simulink model "unknown_case"  (R2021a)
settings: Solver=VariableStepAuto  StartTime=0.0  StopTime=20.0  RelTol=1e-3
libraries: simulink x1
settings Model: Creator=tejal  LastModifiedBy=tejal

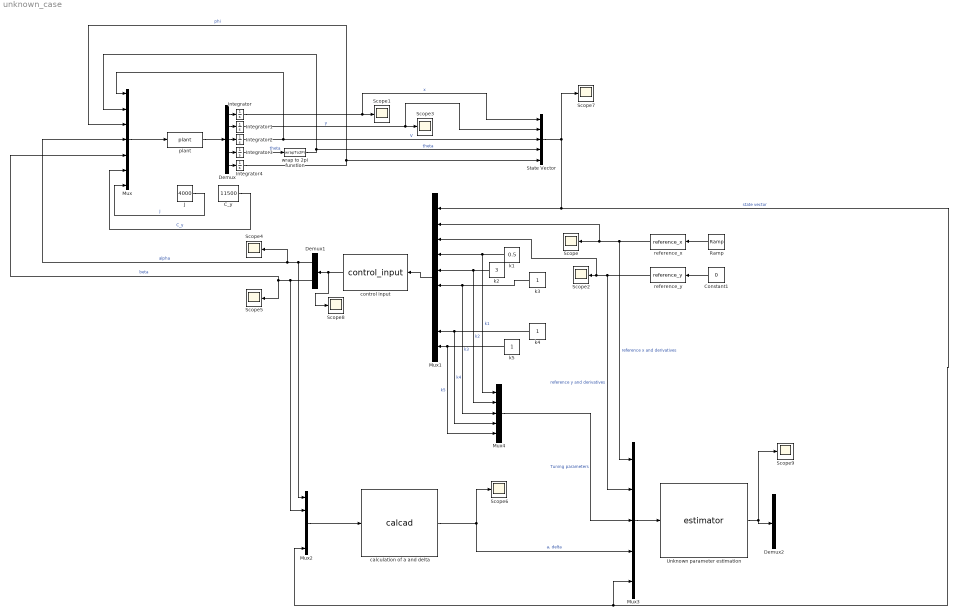
== system unknown_case ==
  C_y : Constant  Value=11500
  Constant1 : Constant  Value=0
  Demux : Demux  Outputs=5
  Demux1 : Demux  Outputs=2
  Demux2 : Demux
  Integrator : Integrator  InitialCondition=1
  Integrator1 : Integrator  InitialCondition=0.00000005
  Integrator2 : Integrator  InitialCondition=1
  Integrator3 : Integrator
  Integrator4 : Integrator
  J : Constant  Value=4000
  Mux : Mux  Inputs=7
  Mux1 : Mux  Inputs=10
  Mux2 : Mux  Inputs=5
  Mux3 : Mux  Inputs=5
  Mux4 : Mux  Inputs=5
  Ramp : simulink/Sources/Ramp  slope=0.3  start=0  InitialOutput=0
  Scope{,1..9} (10 alike) : Scope
  State Vector : Mux  Inputs=5
  Unknown parameter estimation : MATLABFcn  MATLABFcn=estimator  OutputDimensions=4
  calculation of a and delta : MATLABFcn  MATLABFcn=calcad  OutputDimensions=2
  control input : MATLABFcn  MATLABFcn=control_input  OutputDimensions=2
  k1 : Constant  Value=0.5
  k2 : Constant  Value=3
  k3 : Constant
  k4 : Constant
  k5 : Constant
  plant : MATLABFcn  MATLABFcn=plant  OutputDimensions=5
  reference_x : MATLABFcn  MATLABFcn=reference_x  OutputDimensions=4
  reference_y : MATLABFcn  MATLABFcn=reference_y  OutputDimensions=4
  wrap to 2pi function : MATLABFcn  MATLABFcn=wrapTo2Pi
  wires:
  Ramp/1 -> reference_x/1
  reference_x/1 -> Mux3/1, Mux1/2, Scope/1  "reference x and derivatives"
  Constant1/1 -> reference_y/1
  reference_y/1 -> Mux3/2, Mux1/3, Scope2/1  "reference y and derivatives"
  Mux/1 -> plant/1
  plant/1 -> Demux/1
  Demux/1 -> Integrator/1
  Demux/5 -> Integrator4/1
  Demux/4 -> Integrator3/1
  Demux/3 -> Integrator2/1
  Demux/2 -> Integrator1/1
  Integrator/1 -> State Vector/1, Scope1/1  "x"
  Integrator1/1 -> State Vector/2, Scope3/1  "y"
  Integrator2/1 -> Mux/1, State Vector/3  "V"
  Integrator3/1 -> wrap to 2pi function/1  "theta"
  Integrator4/1 -> State Vector/5, Mux/3  "phi"
  J/1 -> Mux/7  "J"
  C_y/1 -> Mux/6  "C_y"
  control input/1 -> Scope8/1, Demux1/1
  Mux1/1 -> control input/1
  State Vector/1 -> Mux3/5, Mux2/5, Mux1/1, Scope7/1  "state vector"
  Demux1/2 -> Mux2/2, Mux/5, Scope5/1  "beta"
  k1/1 -> Mux4/1, Mux1/4  "k1"
  k2/1 -> Mux4/2, Mux1/5  "k2"
  k3/1 -> Mux4/3, Mux1/6  "k3"
  Demux1/1 -> Mux2/1, Scope4/1, Mux/4  "alpha"
  k4/1 -> Mux4/4, Mux1/9  "k4"
  k5/1 -> Mux4/5, Mux1/10  "k5"
  wrap to 2pi function/1 -> State Vector/4, Mux/2  "theta"
  Mux2/1 -> calculation of a and delta/1
  calculation of a and delta/1 -> Mux3/4, Scope6/1  "a, delta"
  Mux3/1 -> Unknown parameter estimation/1
  Mux4/1 -> Mux3/3  "Tuning parameters"
  Unknown parameter estimation/1 -> Scope9/1, Demux2/1
